simulink model "Ablpha_Beta_and_dq_transformations_analysis"  (R2020b)
settings: Solver=FixedStepAuto  StartTime=0.0  StopTime=0.1  FixedStep=1e-5  RelTol=1e-3
PreLoadFcn:
  | va = 1; vb = 1; vc = 1;
  | pa = 0; pb = 120; pc = 240;
  | f = 50;
  | h = 3;
libraries: powerlib_meascontrol x5, simulink x2
settings Model: Creator=arvba41  LastModifiedBy=arvba41

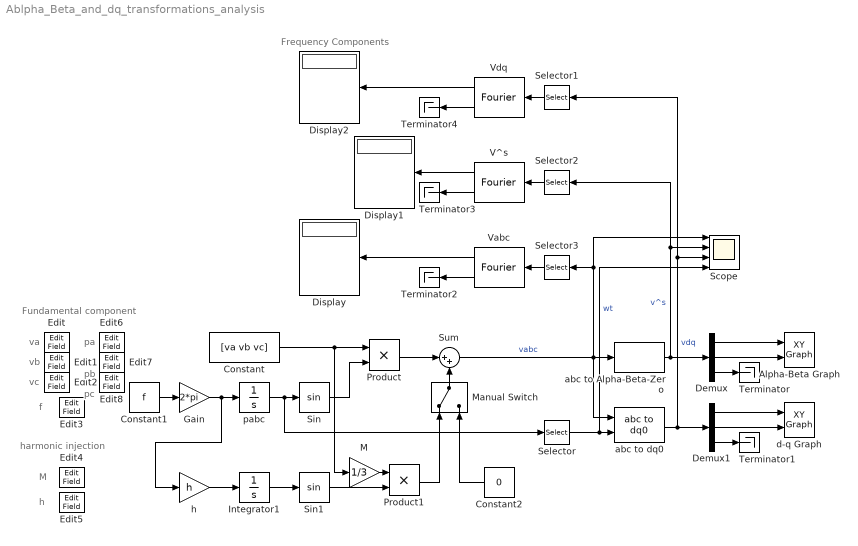
== system Ablpha_Beta_and_dq_transformations_analysis ==
  note: Frequency Components
  note: harmonic injection
  note: va
  note: Fundamental component
  note: vb
  note: vc
  note: f
  note: M
  note: h
  note: pa
  note: pb
  note: pc
  Alpha-Beta Graph : simulink/Sinks/XY Graph  xmin=-2  xmax=2  ymin=-2  ymax=2  st=-1
  Constant : Constant  Value=[va vb vc]
  Constant1 : Constant  Value=f
  Constant2 : Constant  Value=0
  Demux : Demux  Outputs=3
  Demux1 : Demux  Outputs=3
  Display : Display
  Display1 : Display
  Display2 : Display
  Edit{,1..8} (9 alike) : EditField  LabelPosition=Hide  ShowInitialText=on  Alignment=Center
  Gain : Gain  Gain=2*pi
  Integrator1 : Integrator  InitialCondition=deg2rad([pa pb pc])  WrapState=on  WrappedStateUpperValue=2*pi  WrappedStateLowerValue=0
  M : Gain  Gain=1/3
  Manual Switch : ManualSwitch
  Product : Product
  Product1 : Product
  Scope : Scope  NumInputPorts=4
  Selector{,1..3} (4 alike) : Selector  InputPortWidth=3  IndexOptions=Index vector (dialog)  Indices=[1]  OutputSizes=1
  Sin : Trigonometry
  Sin1 : Trigonometry
  Sum : Sum  Inputs=|++
  Terminator{,1..4} (5 alike) : Terminator
  V^s : powerlib_meascontrol/Measurements/Fourier  Freq=f  n=0:h  InInit=[0, 0]  Ts=0
  Vabc : powerlib_meascontrol/Measurements/Fourier  Freq=f  n=0:h  InInit=[0, 0]  Ts=0
  Vdq : powerlib_meascontrol/Measurements/Fourier  Freq=f  n=0:h  InInit=[0, 0]  Ts=0
  abc to Alpha-Beta-Zero : powerlib_meascontrol/Transformations/abc to Alpha-Beta-Zero
  abc to dq0 : powerlib_meascontrol/Transformations/abc to dq0  Alignment=90 degrees behind phase A axis
  d-q Graph : simulink/Sinks/XY Graph  xmin=-2  xmax=2  ymin=-2  ymax=2  st=-1
  h : Gain  Gain=h
  pabc : Integrator  InitialCondition=deg2rad([pa pb pc])  WrapState=on  WrappedStateUpperValue=2*pi  WrappedStateLowerValue=0
  wires:
  Sum/1 -> abc to dq0/1, Selector3/1, Scope/1, abc to Alpha-Beta-Zero/1  "vabc"
  abc to Alpha-Beta-Zero/1 -> Demux/1, Selector2/1, Scope/2  "v^s"
  Demux/1 -> Alpha-Beta Graph/1
  Demux/2 -> Alpha-Beta Graph/2
  Demux/3 -> Terminator/1
  Constant/1 -> M/1, Product/1
  Sin/1 -> Product/2
  Constant1/1 -> Gain/1
  pabc/1 -> Selector/1, Sin/1
  Product/1 -> Sum/1
  Gain/1 -> h/1, pabc/1
  h/1 -> Integrator1/1
  M/1 -> Product1/1
  Integrator1/1 -> Sin1/1
  Product1/1 -> Manual Switch/1
  Manual Switch/1 -> Sum/2
  Constant2/1 -> Manual Switch/2
  Demux1/3 -> Terminator1/1
  Demux1/2 -> d-q Graph/2
  Demux1/1 -> d-q Graph/1
  abc to dq0/1 -> Demux1/1, Selector1/1, Scope/3  "vdq"
  Selector/1 -> Scope/4, abc to dq0/2  "wt"
  Sin1/1 -> Product1/2
  Selector1/1 -> Vdq/1
  Selector2/1 -> V^s/1
  Selector3/1 -> Vabc/1
  Vabc/2 -> Terminator2/1
  V^s/2 -> Terminator3/1
  Vdq/2 -> Terminator4/1
  Vabc/1 -> Display/1
  V^s/1 -> Display1/1
  Vdq/1 -> Display2/1
